simulink model "ADCS_orbiter_detumbling"  (R2022a)
settings: Solver=ode4  StartTime=0.0  StopTime=21085  FixedStep=0.1  MaxStep=1  RelTol=1e-8
values from neighbouring files (symbols this model uses):
  A_cube = 1    [Data_detumbling.m]    (also in main_orbiter_detumbling.m = 12.9)
  A_S2B = [1,0,0;0,-1,0;0,0,-1]    [Data_detumbling.m]
  alpha_x = deg2rad(6/3600)    [Data_detumbling.m]
  alpha_y = deg2rad(6/3600)    [Data_detumbling.m]
  alpha_z = deg2rad(40/3600)    [Data_detumbling.m]
  B_ast = pinv(B)    [Data_detumbling.m]
  ceps = cos(eps)    [Data_detumbling.m]    (also in main_orbiter_detumbling.m)
  F_max = 0.650    (= 0.65)    [Data_detumbling.m]    (also in main_orbiter_detumbling.m = 1.13)
  F_min = 0.160    (= 0.16)    [Data_detumbling.m]    (also in main_orbiter_detumbling.m = 0.19)
  J = [Jx,0,0 ... (first row only)    [Data_detumbling.m]    (also in DisturbanceEvaluation.m = {J_NSO; J_SO}; Thruster_sizing_2.m = diag([12043.36, 15990.19, 8547.84]); main_orbiter.m = J_SO; main_orbiter_detumbling.m = J_SO)
  k_dx = G*J(1,1)/max(diag(J))    [main_orbiter_detumbling.m]
  k_dy = G*J(2,2)/max(diag(J))    [main_orbiter_detumbling.m]
  k_dz = G*J(3,3)/max(diag(J))    [main_orbiter_detumbling.m]
  k_p = 0    [Data_detumbling.m]    (also in main_orbiter_detumbling.m)
  n1 = [1;0;0]    [Data_detumbling.m]    (also in main_orbiter_detumbling.m)
  n2 = [0;1;0]    [Data_detumbling.m]    (also in main_orbiter_detumbling.m)
  n3 = [0;0;1]    [Data_detumbling.m]    (also in main_orbiter_detumbling.m)
  n4 = -n1    [Data_detumbling.m]    (also in main_orbiter_detumbling.m)
  n5 = -n2    [Data_detumbling.m]    (also in main_orbiter_detumbling.m)
  n6 = -n3    [Data_detumbling.m]    (also in main_orbiter_detumbling.m)
  n_sun = 2*pi/(365.25*24*3600)    (= 1.99102127766e-07)    [Data_detumbling.m]    (also in main_orbiter_detumbling.m)
  P = F_e/c    [Data_detumbling.m]    (also in main_orbiter_detumbling.m)
  qbn0 = qrand./norm(qrand)    [main_orbiter.m]    (also in main_orbiter_detumbling.m)
  R = diag([lx_mb/2 ly_mb/2 lz_mb/2]) * [0  0  1  1  0  0 -1 -1 ... (first row only)    [Data_detumbling.m]    (also in main_orbiter_detumbling.m = 0.5*[-ly*cos(inc)              ly*cos(inc)            ly*cos)
  R_ast = pinv(R)    [Data_detumbling.m]    (also in main_orbiter_detumbling.m)
  r_i = r_cube * [n1,n2,n3,n4,n5,n6]    [Data_detumbling.m]    (also in main_orbiter_detumbling.m = [lx/2-cm_off_x  -cm_off_x       -cm_off_x        lx/2+cm_off)
  rho_d = 0.1    [Data_detumbling.m]    (also in main_orbiter_detumbling.m)
  rho_s = 0.5    [Data_detumbling.m]    (also in main_orbiter_detumbling.m)
  S_star1 = S_star1/norm(S_star1)    [Data_detumbling.m]
  S_star2 = S_star2/norm(S_star2)    [Data_detumbling.m]
  S_star3 = S_star3/norm(S_star3)    [Data_detumbling.m]
  S_star4 = S_star4/norm(S_star4)    [Data_detumbling.m]
  seps = sin(eps)    [Data_detumbling.m]    (also in main_orbiter_detumbling.m)
  sigma_ARW = deg2rad(0.001)    [main_orbiter_detumbling.m]
  state0 = [r_vec_new; v_vec_new]    [main_orbiter_detumbling.m]
  w = ones(length(R(1,:)),1)    [Data_detumbling.m]    (also in main_orbiter_detumbling.m)
  w_c = [0 0 0]'    [Data_detumbling.m]    (also in main_orbiter_detumbling.m)
  wb0 = 0.0001*rand(3, 1)    [main_orbiter.m]    (also in main_orbiter_detumbling.m = 0.1*rand(3, 1))
libraries: vrlib x8, matrix_library x1, simulink x1
(part 1 of 3)
settings Model: Creator=pietr  LastModifiedBy=26ele
settings DebuggingCC: UnconnectedInputMsg=warning  UnconnectedOutputMsg=warning  UnconnectedLineMsg=warning
settings RTWCC: DLArmComputeVersion=19.05

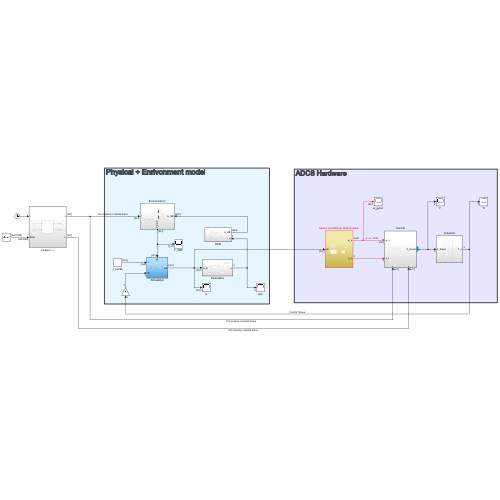
[thumbnail: Simulink's stored preview of the top-level diagram]
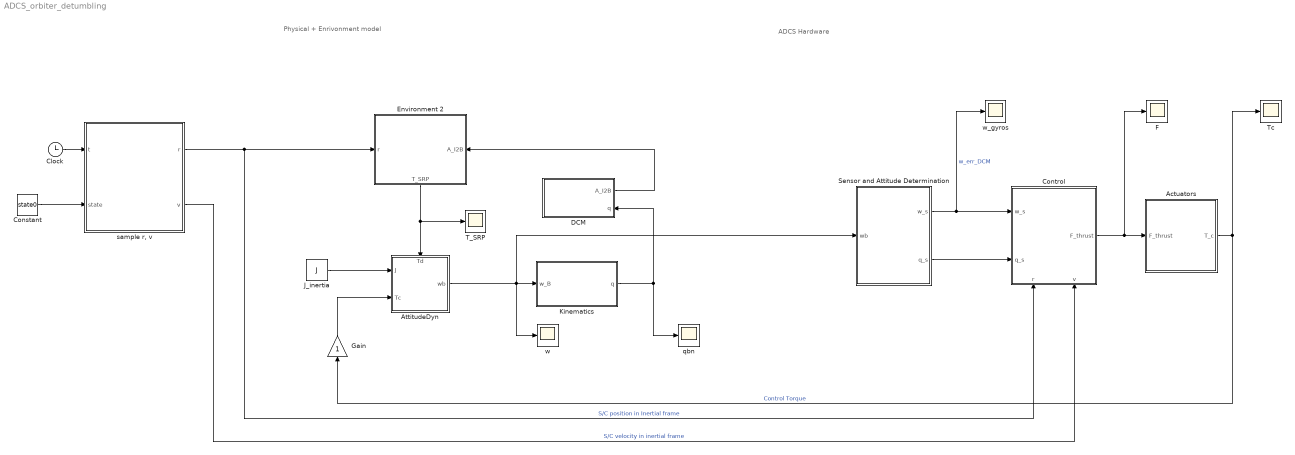
== system ADCS_orbiter_detumbling ==
  note: ADCS Hardware
  note: Physical + Enrivonment model
  Actuators : Subsystem
  AttitudeDyn : Subsystem
      settings: PortSchema="{\"entries\":[{\"content\":{\"sides\":[{\"content\":{\"connectorIds\":[\"In1\",\"In2\"]},\"type\":\"ConnectorPlacement.EquallySpacedRectSide\",\"uuid\":\"958d75f1-056c-4b4d-86fe-843bce156aeb\"},{\"content\":{\"connectorIds\":[\"Out1\"],\"side\":\"RIGHT\"},\"type\":\"ConnectorPlacement.EquallySpacedRectSide\",\"uuid\":\"65b3071b-d244-4f7f-a636-268af73b654f\"},{\"content\":{\"connectorIds\":[\"In3\"],\"side\":\"TOP\"},\"type\":\"ConnectorPlacement.EquallySpacedRectSide\",\"uuid\":\"8fd4fbc8-fd35-4e33-9d82-975bc389520f\"}]},\"type\":\"ConnectorPlacement.EquallySpacedConnector\",\"uuid\":\"8674dee0-aed3-475f-b5bf-17cea7319dbd\"}],\"packageUris\":[\"http://schema.mathworks.com/mf0/Connector/R2020b\"],\"version\":\"1.0\"}"
  Clock : Clock
  Constant : Constant  Value=state0
  Control : Subsystem
      settings: PortSchema="{\"entries\":[{\"content\":{\"sides\":[{\"content\":{\"connectorIds\":[\"In1\",\"In2\"]},\"type\":\"ConnectorPlacement.EquallySpacedRectSide\",\"uuid\":\"b61ecf6f-2766-421f-83dd-a531983edb9b\"},{\"content\":{\"connectorIds\":[\"Out1\"],\"side\":\"RIGHT\"},\"type\":\"ConnectorPlacement.EquallySpacedRectSide\",\"uuid\":\"105d38bf-fae8-4021-992b-3ab993bb750f\"},{\"content\":{\"connectorIds\":[\"In3\",\"In4\"],\"side\":\"TOP\"},\"type\":\"ConnectorPlacement.EquallySpacedRectSide\",\"uuid\":\"14e2d814-54f7-4199-8067-b878a77cfeec\"},{\"content\":{\"connectorIds\":[],\"side\":\"HIDDEN\"},\"type\":\"ConnectorPlacement.EquallySpacedRectSide\",\"uuid\":\"daf11c52-f465-40fd-b237-d971bdc47ecf\"}]},\"type\":\"ConnectorPlacement.EquallySpacedConnector\",\"uuid\":\"1c3e84f7-0d8e-475e-a711-13d0c4ce2024\"}],\"packageUris\":[\"http://schema.mathworks.com/mf0/Connector/R2020b\"],\"version\":\"1.0\"}"
  DCM : Subsystem
      settings: PortSchema="{\"entries\":[{\"content\":{\"sides\":[{\"content\":{\"connectorIds\":[]},\"type\":\"ConnectorPlacement.EquallySpacedRectSide\",\"uuid\":\"a2c03dcc-42ba-46b4-8766-9623140e285d\"},{\"content\":{\"connectorIds\":[\"Out1\",\"In1\"],\"side\":\"RIGHT\"},\"type\":\"ConnectorPlacement.EquallySpacedRectSide\",\"uuid\":\"181415b4-e06f-4a1b-bdae-77d0c2a7a22b\"},{\"content\":{\"connectorIds\":[],\"side\":\"TOP\"},\"type\":\"ConnectorPlacement.EquallySpacedRectSide\",\"uuid\":\"58a9c1ec-db17-43bd-920d-21c7ba7b5be3\"}]},\"type\":\"ConnectorPlacement.EquallySpacedConnector\",\"uuid\":\"76c9aeb0-6471-4cee-b641-2f0ff4597d57\"}],\"packageUris\":[\"http://schema.mathworks.com/mf0/Connector/R2020b\"],\"version\":\"1.0\"}"
  Environment 2 : Subsystem
      settings: PortSchema="{\"entries\":[{\"content\":{\"sides\":[{\"content\":{\"connectorIds\":[\"In1\"]},\"type\":\"ConnectorPlacement.EquallySpacedRectSide\",\"uuid\":\"bd1273ef-f007-48bf-a06f-e15d30a0e351\"},{\"content\":{\"connectorIds\":[\"In2\"],\"side\":\"RIGHT\"},\"type\":\"ConnectorPlacement.EquallySpacedRectSide\",\"uuid\":\"da98429c-d110-4330-bad5-271dcf5066c0\"},{\"content\":{\"connectorIds\":[],\"side\":\"TOP\"},\"type\":\"ConnectorPlacement.EquallySpacedRectSide\",\"uuid\":\"0aff5828-a0c0-41cd-a03e-5c9afd67cac4\"},{\"content\":{\"connectorIds\":[\"Out1\"],\"side\":\"BOTTOM\"},\"type\":\"ConnectorPlacement.EquallySpacedRectSide\",\"uuid\":\"8a284005-ec92-4f7e-b102-e371d7da8945\"}]},\"type\":\"ConnectorPlacement.EquallySpacedConnector\",\"uuid\":\"e9c1be51-430e-49aa-8c1f-f1d04716ab80\"}],\"packageUris\":[\"http://schema.mathworks.com/mf0/Connector/R2020b\"],\"version\":\"1.0\"}"
  F : Scope
  Gain : Gain
  J_inertia : Constant  Value=J  VectorParams1D=off
  Kinematics : Subsystem
  Sensor and Attitude Determination : Subsystem
  T_SRP : Scope
  Tc : Scope
  qbn : Scope
  "sample r, v" : Subsystem
  w : Scope
  w_gyros : Scope
  wires:
  Clock/1 -> "sample r, v"/1(t)
  Constant/1 -> "sample r, v"/2(state)
  "sample r, v"/1(r) -> Environment 2/1(r), Control/3(r)  "S/C position in Inertial frame"
  Kinematics/1(q) -> qbn/1, DCM/1(q)
  Sensor and Attitude Determination/1(w_s) -> w_gyros/1, Control/2(w_s)  "w_err_DCM"
  Sensor and Attitude Determination/2(q_s) -> Control/1(q_s)
  "sample r, v"/2(v) -> Control/4(v)  "S/C velocity in inertial frame"
  Control/1(F_thrust) -> F/1, Actuators/1(F_thrust)
  Actuators/1(T_c) -> Gain/1, Tc/1  "Control Torque"
  Gain/1 -> AttitudeDyn/2(Tc)
  AttitudeDyn/1(wb) -> w/1, Sensor and Attitude Determination/1(wb), Kinematics/1(w_B)
  J_inertia/1 -> AttitudeDyn/1(J)
  DCM/1(A_I2B) -> Environment 2/2(A_I2B)
  Environment 2/1(T_SRP) -> T_SRP/1, AttitudeDyn/3(Td)

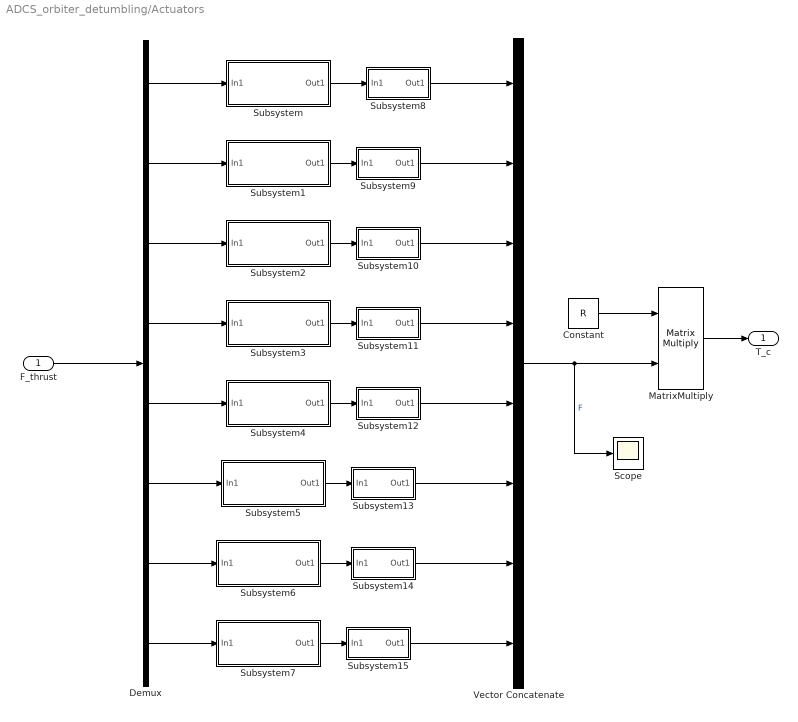
== system ADCS_orbiter_detumbling/Actuators ==
  F_thrust : Inport
  Constant : Constant  Value=R
  Demux : Demux  Outputs=8
  MatrixMultiply : Product  Multiplication=Matrix(*)
  Scope : Scope
  Subsystem : Subsystem
  Subsystem1 : Subsystem
  Subsystem10 : Subsystem
  Subsystem11 : Subsystem
  Subsystem12 : Subsystem
  Subsystem13 : Subsystem
  Subsystem14 : Subsystem
  Subsystem15 : Subsystem
  Subsystem2 : Subsystem
  Subsystem3 : Subsystem
  Subsystem4 : Subsystem
  Subsystem5 : Subsystem
  Subsystem6 : Subsystem
  Subsystem7 : Subsystem
  Subsystem8 : Subsystem
  Subsystem9 : Subsystem
  Vector Concatenate : Concatenate  NumInputs=8
  T_c : Outport
  wires:
  Constant/1 -> MatrixMultiply/1
  MatrixMultiply/1 -> T_c/1
  Vector Concatenate/1 -> Scope/1, MatrixMultiply/2  "F"
  Demux/8 -> Subsystem7/1(In1)
  Demux/7 -> Subsystem6/1(In1)
  F_thrust/1 -> Demux/1
  Demux/6 -> Subsystem5/1(In1)
  Demux/1 -> Subsystem/1(In1)
  Demux/2 -> Subsystem1/1(In1)
  Demux/3 -> Subsystem2/1(In1)
  Demux/4 -> Subsystem3/1(In1)
  Demux/5 -> Subsystem4/1(In1)
  Subsystem2/1(Out1) -> Subsystem10/1(In1)
  Subsystem3/1(Out1) -> Subsystem11/1(In1)
  Subsystem4/1(Out1) -> Subsystem12/1(In1)
  Subsystem5/1(Out1) -> Subsystem13/1(In1)
  Subsystem6/1(Out1) -> Subsystem14/1(In1)
  Subsystem7/1(Out1) -> Subsystem15/1(In1)
  Subsystem/1(Out1) -> Subsystem8/1(In1)
  Subsystem1/1(Out1) -> Subsystem9/1(In1)
  Subsystem15/1(Out1) -> Vector Concatenate/8
  Subsystem14/1(Out1) -> Vector Concatenate/7
  Subsystem13/1(Out1) -> Vector Concatenate/6
  Subsystem12/1(Out1) -> Vector Concatenate/5
  Subsystem11/1(Out1) -> Vector Concatenate/4
  Subsystem10/1(Out1) -> Vector Concatenate/3
  Subsystem9/1(Out1) -> Vector Concatenate/2
  Subsystem8/1(Out1) -> Vector Concatenate/1

== system ADCS_orbiter_detumbling/AttitudeDyn ==
  J : Inport
  Tc : Inport  Port=2
  Td : Inport  Port=3
  Cross Product1 : matrix_library/Cross Product
      settings: SourceProductBaseCode=SL
  Integrator : Integrator  InitialConditionSource=external
  Product : Product  Multiplication=Matrix(*)
  Product1 : Product  Inputs=/  Multiplication=Matrix(*)
  Sum : Sum  Inputs=-++
  To Workspace : ToWorkspace  VariableName=wb  SampleTime=-1
      settings: Save2DSignal=2-D array (concatenate along first dimension)
  wb0 : Constant  Value=wb0  VectorParams1D=off
  wbdot : Product  Multiplication=Matrix(*)
  wb : Outport
  wires:
  Integrator/1 -> wb/1, To Workspace/1, Product/2, Cross Product1/1
  Product/1 -> Cross Product1/2
  Cross Product1/1 -> Sum/1  "wcrossJw"
  J/1 -> Product1/1, Product/1
  wbdot/1 -> Integrator/1
  wb0/1 -> Integrator/2
  Tc/1 -> Sum/3
  Td/1 -> Sum/2
  Product1/1 -> wbdot/1
  Sum/1 -> wbdot/2

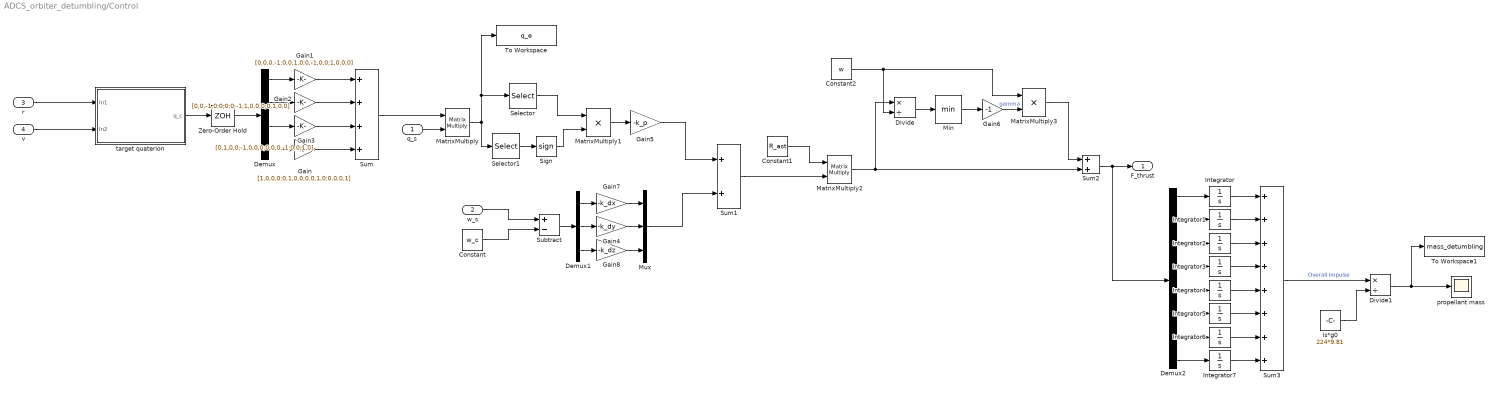
== system ADCS_orbiter_detumbling/Control ==
  q_s : Inport
  w_s : Inport  Port=2
  r : Inport  Port=3
  v : Inport  Port=4
  Constant : Constant  Value=w_c
  Constant1 : Constant  Value=R_ast
  Constant2 : Constant  Value=w
  Demux : Demux
  Demux1 : Demux  Outputs=3
  Demux2 : Demux  Outputs=8
  Divide : Product  Inputs=*/
  Divide1 : Product  Inputs=*/
  Gain : Gain  Gain=[1,0,0,0;0,1,0,0;0,0,1,0;0,0,0,1]
  Gain1 : Gain  Gain=[0,0,0,-1;0,0,1,0;0,-1,0,0;1,0,0,0]
  Gain2 : Gain  Gain=[0,0,-1,0;0,0,0,-1;1,0,0,0;0,1,0,0]
  Gain3 : Gain  Gain=[0,1,0,0;-1,0,0,0;0,0,0,-1;0,0,1,0]
  Gain4 : Gain  Gain=-k_dy
  Gain5 : Gain  Gain=-k_p
  Gain6 : Gain  Gain=-1
  Gain7 : Gain  Gain=-k_dx
  Gain8 : Gain  Gain=-k_dz
  Integrator{,1..7} (8 alike) : Integrator
  Is*g0 : Constant  Value=224*9.81
  MatrixMultiply : Product  Multiplication=Matrix(*)
  MatrixMultiply1 : Product
  MatrixMultiply2 : Product  Multiplication=Matrix(*)
  MatrixMultiply3 : Product
  Min : MinMax
  Mux : Mux  Inputs=3
  Selector : Selector  InputPortWidth=4  IndexOptions=Index vector (dialog)  Indices=[1 2 3]  OutputSizes=1
  Selector1 : Selector  InputPortWidth=4  IndexOptions=Index vector (dialog)  Indices=4  OutputSizes=1
  Sign : Signum
  Subtract : Sum  Inputs=+-
  Sum : Sum  Inputs=++++
  Sum1 : Sum
  Sum2 : Sum
  Sum3 : Sum  Inputs=++++++++
  To Workspace : ToWorkspace  VariableName=q_e  SaveFormat=Timeseries  SampleTime=-1
  To Workspace1 : ToWorkspace  VariableName=mass_detumbling  SampleTime=-1
  Zero-Order Hold : ZeroOrderHold  SampleTime=-1
  propellant mass : Scope
  target quaterion : Subsystem
  F_thrust : Outport
  wires:
  Selector1/1 -> Sign/1
  Constant/1 -> Subtract/2
  Subtract/1 -> Demux1/1
  w_s/1 -> Subtract/1
  MatrixMultiply/1 -> Selector1/1, Selector/1, To Workspace/1
  Zero-Order Hold/1 -> Demux/1
  target quaterion/1(q_c) -> Zero-Order Hold/1
  v/1 -> target quaterion/2(In2)
  r/1 -> target quaterion/1(In1)
  Gain5/1 -> Sum1/1
  Selector/1 -> MatrixMultiply1/1
  MatrixMultiply1/1 -> Gain5/1
  q_s/1 -> MatrixMultiply/2
  Sum/1 -> MatrixMultiply/1
  Gain/1 -> Sum/4
  Gain3/1 -> Sum/3
  Gain2/1 -> Sum/2
  Gain1/1 -> Sum/1
  Demux/2 -> Gain2/1
  Demux/3 -> Gain3/1
  Demux/1 -> Gain1/1
  Demux/4 -> Gain/1
  Sign/1 -> MatrixMultiply1/2
  Sum1/1 -> MatrixMultiply2/2
  Sum2/1 -> Demux2/1, F_thrust/1
  MatrixMultiply2/1 -> Divide/1, Sum2/2
  Divide/1 -> Min/1
  Constant1/1 -> MatrixMultiply2/1
  Gain6/1 -> MatrixMultiply3/2  "gamma"
  Min/1 -> Gain6/1
  Constant2/1 -> MatrixMultiply3/1, Divide/2
  MatrixMultiply3/1 -> Sum2/1
  Demux1/1 -> Gain7/1
  Gain7/1 -> Mux/1
  Demux1/2 -> Gain4/1
  Gain4/1 -> Mux/2
  Demux1/3 -> Gain8/1
  Gain8/1 -> Mux/3
  Mux/1 -> Sum1/2
  Integrator/1 -> Sum3/1
  Demux2/1 -> Integrator/1
  Demux2/2 -> Integrator1/1
  Demux2/8 -> Integrator7/1
  Demux2/7 -> Integrator6/1
  Demux2/6 -> Integrator5/1
  Demux2/5 -> Integrator4/1
  Demux2/4 -> Integrator3/1
  Demux2/3 -> Integrator2/1
  Integrator1/1 -> Sum3/2
  Integrator2/1 -> Sum3/3
  Integrator3/1 -> Sum3/4
  Integrator4/1 -> Sum3/5
  Integrator5/1 -> Sum3/6
  Integrator6/1 -> Sum3/7
  Integrator7/1 -> Sum3/8
  Sum3/1 -> Divide1/1  "Overall Impulse"
  Is*g0/1 -> Divide1/2
  Divide1/1 -> To Workspace1/1, propellant mass/1

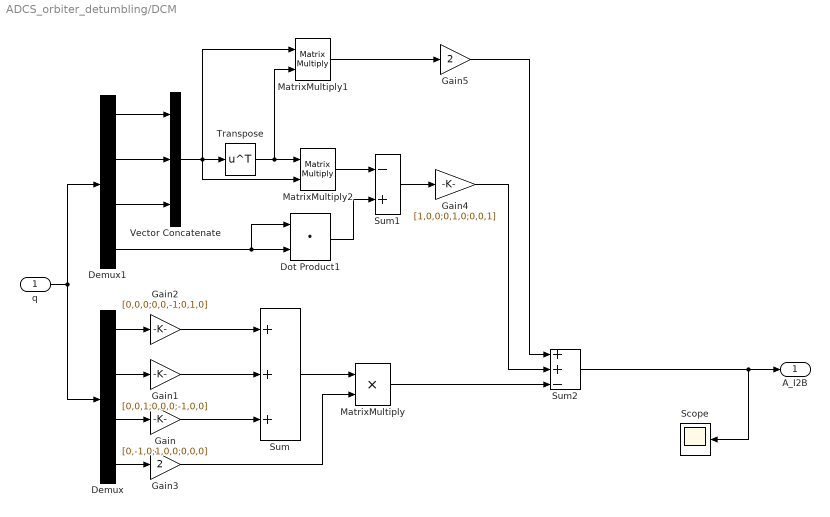
== system ADCS_orbiter_detumbling/DCM ==
  q : Inport
  Demux : Demux
  Demux1 : Demux
  Dot Product1 : DotProduct  OutDataTypeStr=Inherit: Inherit via internal rule
  Gain : Gain  Gain=[0,-1,0;1,0,0;0,0,0]
  Gain1 : Gain  Gain=[0,0,1;0,0,0;-1,0,0]
  Gain2 : Gain  Gain=[0,0,0;0,0,-1;0,1,0]
  Gain3 : Gain  Gain=2
  Gain4 : Gain  Gain=[1,0,0;0,1,0;0,0,1]
  Gain5 : Gain  Gain=2
  MatrixMultiply : Product
  MatrixMultiply1 : Product  Multiplication=Matrix(*)
  MatrixMultiply2 : Product  Multiplication=Matrix(*)
  Scope : Scope
  Sum : Sum  Inputs=+++
  Sum1 : Sum  Inputs=-+
  Sum2 : Sum  Inputs=++-
  Transpose : Math  Operator=transpose
  Vector Concatenate : Concatenate  NumInputs=3
  A_I2B : Outport
  wires:
  q/1 -> Demux/1, Demux1/1
  Demux/3 -> Gain/1
  Demux/2 -> Gain1/1
  Demux/1 -> Gain2/1
  Gain2/1 -> Sum/1
  Gain1/1 -> Sum/2
  Gain/1 -> Sum/3
  Demux/4 -> Gain3/1
  Gain3/1 -> MatrixMultiply/2
  Sum/1 -> MatrixMultiply/1
  Demux1/1 -> Vector Concatenate/1
  Demux1/2 -> Vector Concatenate/2
  Demux1/3 -> Vector Concatenate/3
  Vector Concatenate/1 -> MatrixMultiply1/1, MatrixMultiply2/2, Transpose/1
  Transpose/1 -> MatrixMultiply1/2, MatrixMultiply2/1
  Demux1/4 -> Dot Product1/1, Dot Product1/2
  MatrixMultiply2/1 -> Sum1/1
  Dot Product1/1 -> Sum1/2
  Sum1/1 -> Gain4/1
  MatrixMultiply/1 -> Sum2/3
  Gain4/1 -> Sum2/2
  MatrixMultiply1/1 -> Gain5/1
  Gain5/1 -> Sum2/1
  Sum2/1 -> Scope/1, A_I2B/1

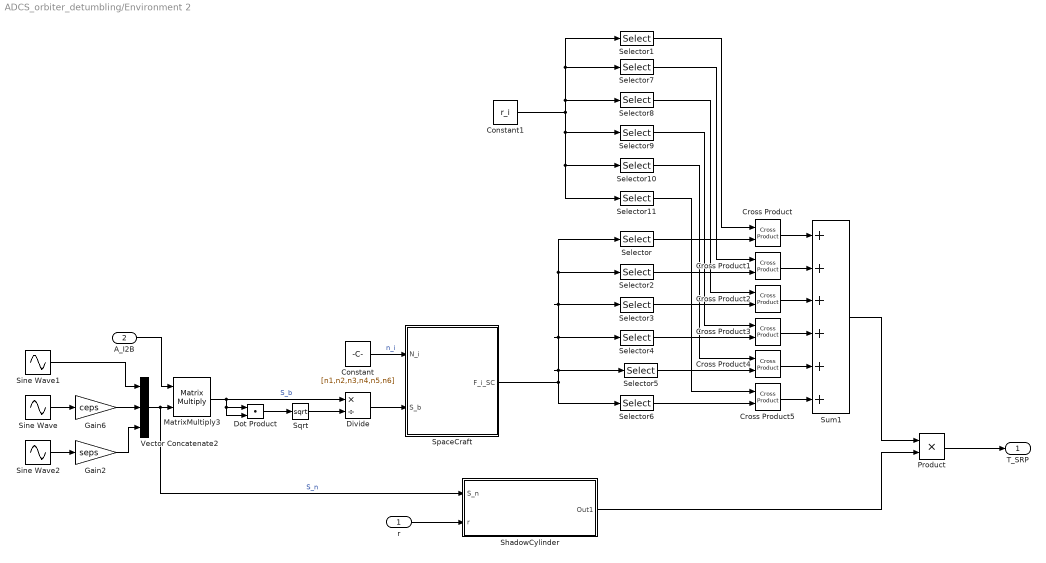
== system ADCS_orbiter_detumbling/Environment 2 ==
  r : Inport
  A_I2B : Inport  Port=2
  Constant : Constant  Value=[n1,n2,n3,n4,n5,n6]
  Constant1 : Constant  Value=r_i  VectorParams1D=off
  Cross Product{,1..5} (6 alike) : vrlib/Utilities/Cross Product
  Divide : Product  Inputs=*/
  Dot Product : DotProduct  OutDataTypeStr=Inherit: Inherit via internal rule
  Gain2 : Gain  Gain=seps
  Gain6 : Gain  Gain=ceps
  MatrixMultiply3 : Product  Multiplication=Matrix(*)
  Product : Product
  Selector : Selector  NumberOfDimensions=2  InputPortWidth=3  IndexOptions=Select all,Index vector (dialog)  Indices=1,1  OutputSizes=1,1
  Selector1 : Selector  NumberOfDimensions=2  InputPortWidth=3  IndexOptions=Select all,Index vector (dialog)  Indices=1,1  OutputSizes=1,1
  Selector10 : Selector  NumberOfDimensions=2  InputPortWidth=3  IndexOptions=Select all,Index vector (dialog)  Indices=5,5  OutputSizes=1,1
  Selector11 : Selector  NumberOfDimensions=2  InputPortWidth=3  IndexOptions=Select all,Index vector (dialog)  Indices=6,6  OutputSizes=1,1
  Selector2 : Selector  NumberOfDimensions=2  InputPortWidth=3  IndexOptions=Select all,Index vector (dialog)  Indices=2,2  OutputSizes=1,1
  Selector3 : Selector  NumberOfDimensions=2  InputPortWidth=3  IndexOptions=Select all,Index vector (dialog)  Indices=3,3  OutputSizes=1,1
  Selector4 : Selector  NumberOfDimensions=2  InputPortWidth=3  IndexOptions=Select all,Index vector (dialog)  Indices=4,4  OutputSizes=1,1
  Selector5 : Selector  NumberOfDimensions=2  InputPortWidth=3  IndexOptions=Select all,Index vector (dialog)  Indices=5,5  OutputSizes=1,1
  Selector6 : Selector  NumberOfDimensions=2  InputPortWidth=3  IndexOptions=Select all,Index vector (dialog)  Indices=6,6  OutputSizes=1,1
  Selector7 : Selector  NumberOfDimensions=2  InputPortWidth=3  IndexOptions=Select all,Index vector (dialog)  Indices=2,2  OutputSizes=1,1
  Selector8 : Selector  NumberOfDimensions=2  InputPortWidth=3  IndexOptions=Select all,Index vector (dialog)  Indices=3,3  OutputSizes=1,1
  Selector9 : Selector  NumberOfDimensions=2  InputPortWidth=3  IndexOptions=Select all,Index vector (dialog)  Indices=4,4  OutputSizes=1,1
  ShadowCylinder : Subsystem
  Sine Wave : Sin  Frequency=n_sun  SampleTime=0
  Sine Wave1 : Sin  Frequency=n_sun  Phase=pi/2  SampleTime=0
  Sine Wave2 : Sin  Frequency=n_sun  SampleTime=0
  SpaceCraft : Subsystem
  Sqrt : Sqrt
  Sum1 : Sum  Inputs=++++++
  Vector Concatenate2 : Concatenate  NumInputs=3
  T_SRP : Outport
  wires:
  SpaceCraft/1(F_i_SC) -> Selector5/1, Selector4/1, Selector3/1, Selector/1, Selector2/1, Selector6/1
  A_I2B/1 -> MatrixMultiply3/1
  Selector10/1 -> Cross Product4/1
  Gain2/1 -> Vector Concatenate2/3
  MatrixMultiply3/1 -> Divide/1, Dot Product/2, Dot Product/1  "S_b"
  Selector11/1 -> Cross Product5/1
  Cross Product2/1 -> Sum1/3
  Selector5/1 -> Cross Product4/2
  Selector9/1 -> Cross Product3/1
  Selector1/1 -> Cross Product/1
  Cross Product5/1 -> Sum1/6
  Sine Wave2/1 -> Gain2/1
  Dot Product/1 -> Sqrt/1
  Cross Product4/1 -> Sum1/5
  Selector6/1 -> Cross Product5/2
  Cross Product3/1 -> Sum1/4
  Selector4/1 -> Cross Product3/2
  Cross Product/1 -> Sum1/1
  Constant/1 -> SpaceCraft/1(N_i)  "n_i"
  Divide/1 -> SpaceCraft/2(S_b)
  Selector2/1 -> Cross Product1/2
  Selector8/1 -> Cross Product2/1
  Cross Product1/1 -> Sum1/2
  Selector3/1 -> Cross Product2/2
  Selector7/1 -> Cross Product1/1
  Selector/1 -> Cross Product/2
  Gain6/1 -> Vector Concatenate2/2
  Sine Wave/1 -> Gain6/1
  Sine Wave1/1 -> Vector Concatenate2/1
  Sum1/1 -> Product/1
  Sqrt/1 -> Divide/2
  Vector Concatenate2/1 -> ShadowCylinder/1(S_n), MatrixMultiply3/2  "S_n"
  r/1 -> ShadowCylinder/2(r)
  ShadowCylinder/1(Out1) -> Product/2
  Product/1 -> T_SRP/1
  Constant1/1 -> Selector1/1, Selector7/1, Selector8/1, Selector10/1, Selector11/1, Selector9/1

== system ADCS_orbiter_detumbling/Kinematics ==
  w_B : Inport
  Derivative : Derivative
  Quaternion : Subsystem
  To Workspace : ToWorkspace  VariableName=q  SampleTime=-1
  To Workspace1 : ToWorkspace  VariableName=w_B_dot  SaveFormat=Timeseries  SampleTime=-1
  q : Outport
  wires:
  Quaternion/1(q) -> To Workspace/1, q/1
  w_B/1 -> Derivative/1, Quaternion/1(w_B)
  Derivative/1 -> To Workspace1/1

== system ADCS_orbiter_detumbling/Sensor and Attitude Determination ==
  wb : Inport
  Gyroscope1 : Subsystem
  Star Trackers1 : Subsystem  Commented=on
  Subsystem2 : Subsystem
  Subsystem3 : Subsystem
  Subsystem4 : Subsystem
  Terminator : Terminator
  Terminator1 : Terminator
  w_s : Outport
  q_s : Outport  Port=2
  wires:
  Subsystem2/1(qerr) -> q_s/1
  Gyroscope1/1(w_GYR) -> w_s/1, Subsystem2/1(w_GYR)
  Star Trackers1/1(A_I2B_err) -> Subsystem4/1(A_I2B_err), Subsystem3/1(A_I2B_err)
  Subsystem3/1(qerr) -> Terminator1/1
  Subsystem4/1(w_err_DCM) -> Terminator/1
  wb/1 -> Gyroscope1/1(w)

== system ADCS_orbiter_detumbling/sample r, v ==
  t : Inport
  state : Inport  Port=2
  MATLAB Function : MATLAB Function  TreatAsAtomicUnit=on
  r : Outport
  v : Outport  Port=2
  wires:
  t/1 -> MATLAB Function/1(t)
  state/1 -> MATLAB Function/2(A)
  MATLAB Function/1(r) -> r/1
  MATLAB Function/2(v) -> v/1

== system ADCS_orbiter_detumbling/Actuators/Subsystem ==
  In1 : Inport
  Constant : Constant  Value=F_max
  Constant1 : Constant  Value=0
  If : If  IfExpression=u1 > F_max  ElseIfExpressions=u1<F_min
  If Action Subsystem : Subsystem  TreatAsAtomicUnit=on
  If Action Subsystem1 : Subsystem  TreatAsAtomicUnit=on
  If Action Subsystem2 : Subsystem  TreatAsAtomicUnit=on
  Merge : Merge  Inputs=3
  Out1 : Outport
  wires:
  In1/1 -> If/1, If Action Subsystem2/1(In1)
  If/1 -> If Action Subsystem/Action
  Constant/1 -> If Action Subsystem/1(In1)
  Constant1/1 -> If Action Subsystem1/1(In1)
  If/2 -> If Action Subsystem1/Action
  If/3 -> If Action Subsystem2/Action
  If Action Subsystem2/1(Out1) -> Merge/3
  If Action Subsystem/1(Out1) -> Merge/1
  If Action Subsystem1/1(Out1) -> Merge/2
  Merge/1 -> Out1/1

== system ADCS_orbiter_detumbling/Actuators/Subsystem1 ==
  In1 : Inport
  Constant : Constant  Value=F_max
  Constant1 : Constant  Value=0
  If : If  IfExpression=u1 > F_max  ElseIfExpressions=u1<F_min
  If Action Subsystem : Subsystem  TreatAsAtomicUnit=on
  If Action Subsystem1 : Subsystem  TreatAsAtomicUnit=on
  If Action Subsystem2 : Subsystem  TreatAsAtomicUnit=on
  Merge : Merge  Inputs=3
  Out1 : Outport
  wires:
  In1/1 -> If Action Subsystem2/1(In1), If/1
  If/1 -> If Action Subsystem/Action
  Constant/1 -> If Action Subsystem/1(In1)
  Constant1/1 -> If Action Subsystem1/1(In1)
  If/2 -> If Action Subsystem1/Action
  If/3 -> If Action Subsystem2/Action
  If Action Subsystem2/1(Out1) -> Merge/3
  If Action Subsystem/1(Out1) -> Merge/1
  If Action Subsystem1/1(Out1) -> Merge/2
  Merge/1 -> Out1/1

== system ADCS_orbiter_detumbling/Actuators/Subsystem10 ==
  In1 : Inport
  Delay : Delay  DelayLength=1
  Delay1 : Delay
  If : If
  If Action Subsystem : Subsystem  TreatAsAtomicUnit=on
  If Action Subsystem1 : Subsystem  TreatAsAtomicUnit=on
  Merge : Merge
  Out1 : Outport
  wires:
  In1/1 -> Delay/1, Delay1/1, If Action Subsystem1/1(In1), If Action Subsystem/1(In1), If/1
  If/1 -> If Action Subsystem/Action
  If/2 -> If Action Subsystem1/Action
  If Action Subsystem/1(Out2) -> Merge/1  "u"
  If Action Subsystem1/1(Out1) -> Merge/2  "u"
  Merge/1 -> Out1/1
  Delay/1 -> If Action Subsystem1/2(Input)
  Delay1/1 -> If Action Subsystem1/3(Input1)

== system ADCS_orbiter_detumbling/Actuators/Subsystem11 ==
  In1 : Inport
  Delay : Delay  DelayLength=1
  Delay1 : Delay
  If : If
  If Action Subsystem : Subsystem  TreatAsAtomicUnit=on
  If Action Subsystem1 : Subsystem  TreatAsAtomicUnit=on
  Merge : Merge
  Out1 : Outport
  wires:
  Delay1/1 -> If Action Subsystem1/3(Input1)
  Delay/1 -> If Action Subsystem1/2(Input)
  Merge/1 -> Out1/1
  If Action Subsystem1/1(Out1) -> Merge/2  "u"
  If Action Subsystem/1(Out2) -> Merge/1  "u"
  If/2 -> If Action Subsystem1/Action
  If/1 -> If Action Subsystem/Action
  In1/1 -> If/1, If Action Subsystem/1(In1), If Action Subsystem1/1(In1), Delay1/1, Delay/1

== system ADCS_orbiter_detumbling/Actuators/Subsystem12 ==
  In1 : Inport
  Delay : Delay  DelayLength=1
  Delay1 : Delay
  If : If
  If Action Subsystem : Subsystem  TreatAsAtomicUnit=on
  If Action Subsystem1 : Subsystem  TreatAsAtomicUnit=on
  Merge : Merge
  Out1 : Outport
  wires:
  In1/1 -> Delay/1, Delay1/1, If Action Subsystem1/1(In1), If Action Subsystem/1(In1), If/1
  If/1 -> If Action Subsystem/Action
  If/2 -> If Action Subsystem1/Action
  If Action Subsystem/1(Out2) -> Merge/1  "u"
  If Action Subsystem1/1(Out1) -> Merge/2  "u"
  Merge/1 -> Out1/1
  Delay/1 -> If Action Subsystem1/2(Input)
  Delay1/1 -> If Action Subsystem1/3(Input1)

== system ADCS_orbiter_detumbling/Actuators/Subsystem13 ==
  In1 : Inport
  Delay : Delay  DelayLength=1
  Delay1 : Delay
  If : If
  If Action Subsystem : Subsystem  TreatAsAtomicUnit=on
  If Action Subsystem1 : Subsystem  TreatAsAtomicUnit=on
  Merge : Merge
  Scope : Scope  NumInputPorts=2
  Out1 : Outport
  wires:
  Delay1/1 -> If Action Subsystem1/3(Input1)
  Delay/1 -> If Action Subsystem1/2(Input)
  Merge/1 -> Scope/2, Out1/1
  If Action Subsystem1/1(Out1) -> Merge/2  "u"
  If Action Subsystem/1(Out2) -> Merge/1  "u"
  If/2 -> If Action Subsystem1/Action
  If/1 -> If Action Subsystem/Action
  In1/1 -> If/1, Scope/1, If Action Subsystem/1(In1), If Action Subsystem1/1(In1), Delay1/1, Delay/1

== system ADCS_orbiter_detumbling/Actuators/Subsystem14 ==
  In1 : Inport
  Delay : Delay  DelayLength=1
  Delay1 : Delay
  If : If
  If Action Subsystem : Subsystem  TreatAsAtomicUnit=on
  If Action Subsystem1 : Subsystem  TreatAsAtomicUnit=on
  Merge : Merge
  Scope : Scope  NumInputPorts=2
  Out1 : Outport
  wires:
  In1/1 -> Delay/1, Delay1/1, If Action Subsystem1/1(In1), Scope/1, If Action Subsystem/1(In1), If/1
  If/1 -> If Action Subsystem/Action
  If/2 -> If Action Subsystem1/Action
  If Action Subsystem/1(Out2) -> Merge/1  "u"
  If Action Subsystem1/1(Out1) -> Merge/2  "u"
  Merge/1 -> Scope/2, Out1/1
  Delay/1 -> If Action Subsystem1/2(Input)
  Delay1/1 -> If Action Subsystem1/3(Input1)

== system ADCS_orbiter_detumbling/Actuators/Subsystem15 ==
  In1 : Inport
  Delay : Delay  DelayLength=1
  Delay1 : Delay
  If : If
  If Action Subsystem : Subsystem  TreatAsAtomicUnit=on
  If Action Subsystem1 : Subsystem  TreatAsAtomicUnit=on
  Merge : Merge
  Out1 : Outport
  wires:
  Delay1/1 -> If Action Subsystem1/3(Input1)
  Delay/1 -> If Action Subsystem1/2(Input)
  Merge/1 -> Out1/1
  If Action Subsystem1/1(Out1) -> Merge/2  "u"
  If Action Subsystem/1(Out2) -> Merge/1  "u"
  If/2 -> If Action Subsystem1/Action
  If/1 -> If Action Subsystem/Action
  In1/1 -> If/1, If Action Subsystem/1(In1), If Action Subsystem1/1(In1), Delay1/1, Delay/1

== system ADCS_orbiter_detumbling/Actuators/Subsystem2 ==
  In1 : Inport
  Constant : Constant  Value=F_max
  Constant1 : Constant  Value=0
  If : If  IfExpression=u1 > F_max  ElseIfExpressions=u1<F_min
  If Action Subsystem : Subsystem  TreatAsAtomicUnit=on
  If Action Subsystem1 : Subsystem  TreatAsAtomicUnit=on
  If Action Subsystem2 : Subsystem  TreatAsAtomicUnit=on
  Merge : Merge  Inputs=3
  Out1 : Outport
  wires:
  Merge/1 -> Out1/1
  If Action Subsystem1/1(Out1) -> Merge/2
  If Action Subsystem/1(Out1) -> Merge/1
  If Action Subsystem2/1(Out1) -> Merge/3
  If/3 -> If Action Subsystem2/Action
  If/2 -> If Action Subsystem1/Action
  Constant1/1 -> If Action Subsystem1/1(In1)
  Constant/1 -> If Action Subsystem/1(In1)
  If/1 -> If Action Subsystem/Action
  In1/1 -> If/1, If Action Subsystem2/1(In1)

== system ADCS_orbiter_detumbling/Actuators/Subsystem3 ==
  In1 : Inport
  Constant : Constant  Value=F_max
  Constant1 : Constant  Value=0
  If : If  IfExpression=u1 > F_max  ElseIfExpressions=u1<F_min
  If Action Subsystem : Subsystem  TreatAsAtomicUnit=on
  If Action Subsystem1 : Subsystem  TreatAsAtomicUnit=on
  If Action Subsystem2 : Subsystem  TreatAsAtomicUnit=on
  Merge : Merge  Inputs=3
  Out1 : Outport
  wires:
  In1/1 -> If Action Subsystem2/1(In1), If/1
  If/1 -> If Action Subsystem/Action
  Constant/1 -> If Action Subsystem/1(In1)
  Constant1/1 -> If Action Subsystem1/1(In1)
  If/2 -> If Action Subsystem1/Action
  If/3 -> If Action Subsystem2/Action
  If Action Subsystem2/1(Out1) -> Merge/3
  If Action Subsystem/1(Out1) -> Merge/1
  If Action Subsystem1/1(Out1) -> Merge/2
  Merge/1 -> Out1/1

== system ADCS_orbiter_detumbling/Actuators/Subsystem4 ==
  In1 : Inport
  Constant : Constant  Value=F_max
  Constant1 : Constant  Value=0
  If : If  IfExpression=u1 > F_max  ElseIfExpressions=u1<F_min
  If Action Subsystem : Subsystem  TreatAsAtomicUnit=on
  If Action Subsystem1 : Subsystem  TreatAsAtomicUnit=on
  If Action Subsystem2 : Subsystem  TreatAsAtomicUnit=on
  Merge : Merge  Inputs=3
  Out1 : Outport
  wires:
  Merge/1 -> Out1/1
  If Action Subsystem1/1(Out1) -> Merge/2
  If Action Subsystem/1(Out1) -> Merge/1
  If Action Subsystem2/1(Out1) -> Merge/3
  If/3 -> If Action Subsystem2/Action
  If/2 -> If Action Subsystem1/Action
  Constant1/1 -> If Action Subsystem1/1(In1)
  Constant/1 -> If Action Subsystem/1(In1)
  If/1 -> If Action Subsystem/Action
  In1/1 -> If/1, If Action Subsystem2/1(In1)

== system ADCS_orbiter_detumbling/Actuators/Subsystem5 ==
  In1 : Inport
  Constant : Constant  Value=F_max
  Constant1 : Constant  Value=0
  If : If  IfExpression=u1 > F_max  ElseIfExpressions=u1<F_min
  If Action Subsystem : Subsystem  TreatAsAtomicUnit=on
  If Action Subsystem1 : Subsystem  TreatAsAtomicUnit=on
  If Action Subsystem2 : Subsystem  TreatAsAtomicUnit=on
  Merge : Merge  Inputs=3
  Out1 : Outport
  wires:
  In1/1 -> If Action Subsystem2/1(In1), If/1
  If/1 -> If Action Subsystem/Action
  Constant/1 -> If Action Subsystem/1(In1)
  Constant1/1 -> If Action Subsystem1/1(In1)
  If/2 -> If Action Subsystem1/Action
  If/3 -> If Action Subsystem2/Action
  If Action Subsystem2/1(Out1) -> Merge/3
  If Action Subsystem/1(Out1) -> Merge/1
  If Action Subsystem1/1(Out1) -> Merge/2
  Merge/1 -> Out1/1

== system ADCS_orbiter_detumbling/Actuators/Subsystem6 ==
  In1 : Inport
  Constant : Constant  Value=F_max
  Constant1 : Constant  Value=0
  If : If  IfExpression=u1 > F_max  ElseIfExpressions=u1<F_min
  If Action Subsystem : Subsystem  TreatAsAtomicUnit=on
  If Action Subsystem1 : Subsystem  TreatAsAtomicUnit=on
  If Action Subsystem2 : Subsystem  TreatAsAtomicUnit=on
  Merge : Merge  Inputs=3
  Out1 : Outport
  wires:
  Merge/1 -> Out1/1
  If Action Subsystem1/1(Out1) -> Merge/2
  If Action Subsystem/1(Out1) -> Merge/1
  If Action Subsystem2/1(Out1) -> Merge/3
  If/3 -> If Action Subsystem2/Action
  If/2 -> If Action Subsystem1/Action
  Constant1/1 -> If Action Subsystem1/1(In1)
  Constant/1 -> If Action Subsystem/1(In1)
  If/1 -> If Action Subsystem/Action
  In1/1 -> If/1, If Action Subsystem2/1(In1)

== system ADCS_orbiter_detumbling/Actuators/Subsystem7 ==
  In1 : Inport
  Constant : Constant  Value=F_max
  Constant1 : Constant  Value=0
  If : If  IfExpression=u1 > F_max  ElseIfExpressions=u1<F_min
  If Action Subsystem : Subsystem  TreatAsAtomicUnit=on
  If Action Subsystem1 : Subsystem  TreatAsAtomicUnit=on
  If Action Subsystem2 : Subsystem  TreatAsAtomicUnit=on
  Merge : Merge  Inputs=3
  Out1 : Outport
  wires:
  In1/1 -> If Action Subsystem2/1(In1), If/1
  If/1 -> If Action Subsystem/Action
  Constant/1 -> If Action Subsystem/1(In1)
  Constant1/1 -> If Action Subsystem1/1(In1)
  If/2 -> If Action Subsystem1/Action
  If/3 -> If Action Subsystem2/Action
  If Action Subsystem2/1(Out1) -> Merge/3
  If Action Subsystem/1(Out1) -> Merge/1
  If Action Subsystem1/1(Out1) -> Merge/2
  Merge/1 -> Out1/1

== system ADCS_orbiter_detumbling/Actuators/Subsystem8 ==
  In1 : Inport
  Delay : Delay  DelayLength=1
  Delay1 : Delay
  If : If
  If Action Subsystem : Subsystem  TreatAsAtomicUnit=on
  If Action Subsystem1 : Subsystem  TreatAsAtomicUnit=on
  Merge : Merge
  Out1 : Outport
  wires:
  In1/1 -> Delay/1, Delay1/1, If Action Subsystem1/1(In1), If Action Subsystem/1(In1), If/1
  If/1 -> If Action Subsystem/Action
  If/2 -> If Action Subsystem1/Action
  If Action Subsystem/1(Out2) -> Merge/1  "u"
  If Action Subsystem1/1(Out1) -> Merge/2  "u"
  Merge/1 -> Out1/1
  Delay/1 -> If Action Subsystem1/2(Input)
  Delay1/1 -> If Action Subsystem1/3(Input1)

== system ADCS_orbiter_detumbling/Actuators/Subsystem9 ==
  In1 : Inport
  Delay : Delay  DelayLength=1
  Delay1 : Delay
  If : If
  If Action Subsystem : Subsystem  TreatAsAtomicUnit=on
  If Action Subsystem1 : Subsystem  TreatAsAtomicUnit=on
  Merge : Merge
  Out1 : Outport
  wires:
  Delay1/1 -> If Action Subsystem1/3(Input1)
  Delay/1 -> If Action Subsystem1/2(Input)
  Merge/1 -> Out1/1
  If Action Subsystem1/1(Out1) -> Merge/2  "u"
  If Action Subsystem/1(Out2) -> Merge/1  "u"
  If/2 -> If Action Subsystem1/Action
  If/1 -> If Action Subsystem/Action
  In1/1 -> If/1, If Action Subsystem/1(In1), If Action Subsystem1/1(In1), Delay1/1, Delay/1

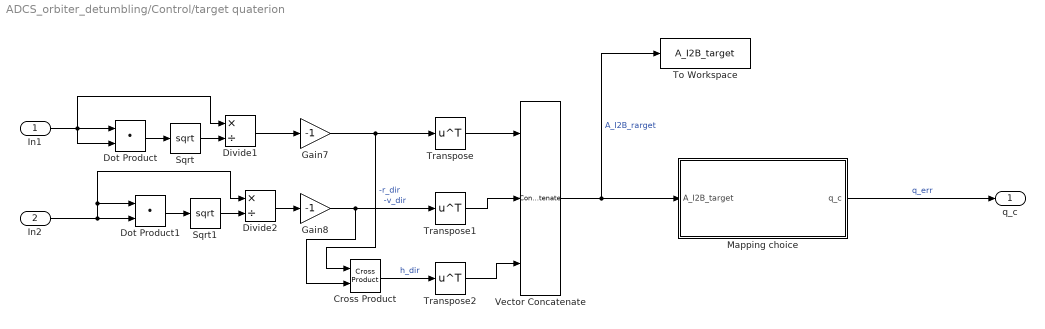
== system ADCS_orbiter_detumbling/Control/target quaterion ==
  In1 : Inport
  In2 : Inport  Port=2
  Cross Product : vrlib/Utilities/Cross Product
  Divide1 : Product  Inputs=*/
  Divide2 : Product  Inputs=*/
  Dot Product : DotProduct  OutDataTypeStr=Inherit: Inherit via internal rule
  Dot Product1 : DotProduct  OutDataTypeStr=Inherit: Inherit via internal rule
  Gain7 : Gain  Gain=-1
  Gain8 : Gain  Gain=-1
  Mapping choice : Subsystem
  Sqrt : Sqrt
  Sqrt1 : Sqrt
  To Workspace : ToWorkspace  VariableName=A_I2B_target  SampleTime=-1
  Transpose : Math  Operator=transpose
  Transpose1 : Math  Operator=transpose
  Transpose2 : Math  Operator=transpose
  Vector Concatenate : Concatenate  NumInputs=3  Mode=Multidimensional array
  q_c : Outport
  wires:
  Mapping choice/1(q_c) -> q_c/1  "q_err"
  Sqrt/1 -> Divide1/2
  Transpose2/1 -> Vector Concatenate/3
  Cross Product/1 -> Transpose2/1  "h_dir"
  Dot Product1/1 -> Sqrt1/1
  Divide2/1 -> Gain8/1
  Sqrt1/1 -> Divide2/2
  Divide1/1 -> Gain7/1
  Vector Concatenate/1 -> To Workspace/1, Mapping choice/1(A_I2B_target)  "A_I2B_rarget"
  Transpose1/1 -> Vector Concatenate/2
  In1/1 -> Dot Product/2, Divide1/1, Dot Product/1
  Gain7/1 -> Transpose/1, Cross Product/1  "-r_dir"
  Dot Product/1 -> Sqrt/1
  Transpose/1 -> Vector Concatenate/1
  In2/1 -> Dot Product1/2, Divide2/1, Dot Product1/1
  Gain8/1 -> Transpose1/1, Cross Product/2  "-v_dir"

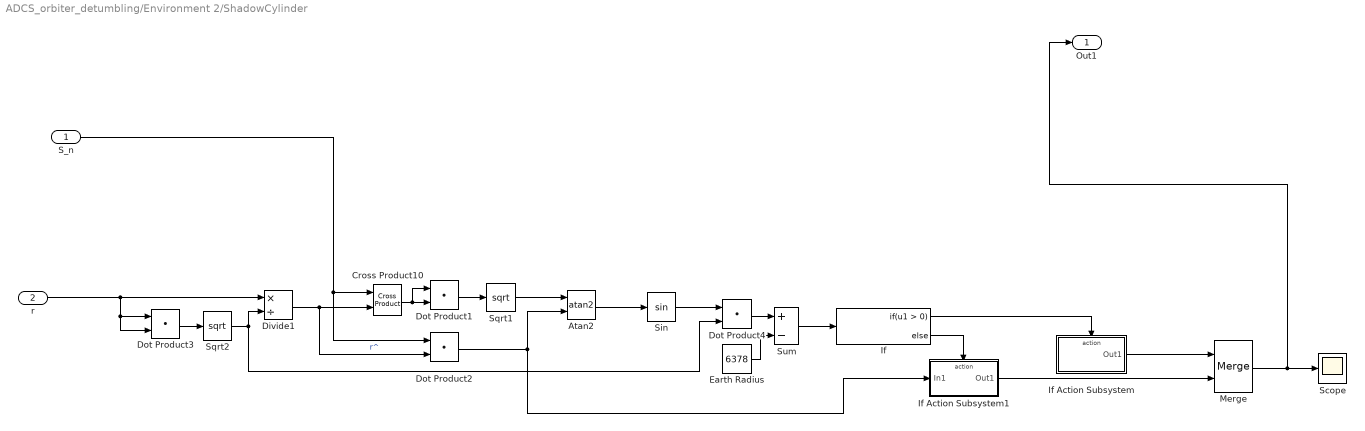
== system ADCS_orbiter_detumbling/Environment 2/ShadowCylinder ==
  S_n : Inport
  r : Inport  Port=2
  Atan2 : Trigonometry  Operator=atan2  OutputSignalType=real
  Cross Product10 : vrlib/Utilities/Cross Product
  Divide1 : Product  Inputs=*/
  Dot Product{1..4} (4 alike) : DotProduct  OutDataTypeStr=Inherit: Inherit via internal rule
  Earth Radius : Constant  Value=6378
  If : If
  If Action Subsystem : Subsystem  TreatAsAtomicUnit=on
  If Action Subsystem1 : Subsystem  TreatAsAtomicUnit=on
  Merge : Merge
  Scope : Scope
  Sin : Trigonometry
  Sqrt1 : Sqrt
  Sqrt2 : Sqrt
  Sum : Sum  Inputs=+-
  Out1 : Outport
  wires:
  Sqrt1/1 -> Atan2/1
  Cross Product10/1 -> Dot Product1/1, Dot Product1/2
  Dot Product1/1 -> Sqrt1/1
  Sqrt2/1 -> Dot Product4/2, Divide1/2
  If/2 -> If Action Subsystem1/Action
  Divide1/1 -> Dot Product2/2, Cross Product10/2  "r^"
  Atan2/1 -> Sin/1
  r/1 -> Divide1/1, Dot Product3/1, Dot Product3/2
  Dot Product2/1 -> If Action Subsystem1/1(In1), Atan2/2
  S_n/1 -> Dot Product2/1, Cross Product10/1
  Sum/1 -> If/1
  Dot Product4/1 -> Sum/1
  If/1 -> If Action Subsystem/Action
  If Action Subsystem/1(Out1) -> Merge/1
  Earth Radius/1 -> Sum/2
  Sin/1 -> Dot Product4/1
  Dot Product3/1 -> Sqrt2/1
  If Action Subsystem1/1(Out1) -> Merge/2
  Merge/1 -> Out1/1, Scope/1

== system ADCS_orbiter_detumbling/Environment 2/SpaceCraft ==
  N_i : Inport
  S_b : Inport  Port=2
  Constant : Constant  Value=2/3*rho_d
  Gain : Gain  Gain=1-rho_s
  Gain1 : Gain  Gain=2*rho_s
  Gain2 : Gain  Gain=-P*A_cube
  Gain3 : Gain  Gain=[1,1,1,1,1,1]
  MatrixMultiply : Product  Multiplication=Matrix(*)
  MatrixMultiply1 : Product  Multiplication=Matrix(*)
  MatrixMultiply2 : Product  Multiplication=Matrix(*)
  Sum : Sum
  Sum1 : Sum
  Transpose : Math  Operator=transpose
  Transpose2 : Math  Operator=transpose
  Zero_If_Negative : Subsystem
  F_i_SC : Outport
  wires:
  N_i/1 -> MatrixMultiply1/1, MatrixMultiply/2  "N_i"
  S_b/1 -> Gain/1, Transpose2/1
  MatrixMultiply/1 -> Gain1/1, Zero_If_Negative/1(In1)  "S_bN_i"
  Gain2/1 -> F_i_SC/1  "F_i_SC"
  Sum/1 -> MatrixMultiply1/2
  MatrixMultiply1/1 -> Sum1/2
  Gain/1 -> Sum1/1
  Sum1/1 -> MatrixMultiply2/1
  MatrixMultiply2/1 -> Gain2/1
  Transpose2/1 -> MatrixMultiply/1
  Gain1/1 -> Transpose/1
  Constant/1 -> Gain3/1
  Gain3/1 -> Sum/2
  Transpose/1 -> Sum/1
  Zero_If_Negative/1(Out1) -> MatrixMultiply2/2

== system ADCS_orbiter_detumbling/Kinematics/Quaternion ==
  w_B : Inport
  Demux : Demux  Outputs=3
  Divide : Product  Inputs=*/
  Dot Product : DotProduct  OutDataTypeStr=Inherit: Inherit via internal rule
  Gain2 : Gain  Gain=1/2
  Gain3 : Gain  Gain=[0,0,0,1;0,0,1,0;0,-1,0,0;-1,0,0,0]
  Gain4 : Gain  Gain=[0,0,-1,0;0,0,0,1;1,0,0,0;0,-1,0,0]
  Gain5 : Gain  Gain=[0,1,0,0;-1,0,0,0;0,0,0,1;0,0,-1,0]
  Integrator1 : Integrator  InitialCondition=qbn0
  MatrixMultiply : Product  Multiplication=Matrix(*)
  Sqrt : Sqrt
  Sum : Sum  Inputs=+++
  q : Outport
  wires:
  Gain4/1 -> Sum/2
  w_B/1 -> Demux/1
  Gain5/1 -> Sum/3
  Demux/2 -> Gain4/1
  Demux/1 -> Gain3/1
  Integrator1/1 -> Dot Product/2, Dot Product/1, Divide/1, q/1  "q"
  Gain3/1 -> Sum/1
  Demux/3 -> Gain5/1
  Gain2/1 -> Integrator1/1
  Sum/1 -> MatrixMultiply/1  "OMEGA"
  Divide/1 -> MatrixMultiply/2  "q"
  MatrixMultiply/1 -> Gain2/1
  Dot Product/1 -> Sqrt/1
  Sqrt/1 -> Divide/2

== system ADCS_orbiter_detumbling/Sensor and Attitude Determination/Gyroscope1 ==
  w : Inport
  Add : Sum  Inputs=+++
  Integrator2 : Integrator
  Mux : Mux  Inputs=3
  Mux1 : Mux  Inputs=3
  Random Number{,1..5} (6 alike) : RandomNumber  Variance=sigma_ARW^2  Seed=20  SampleTime=0.1
  Zero-Order Hold : ZeroOrderHold  SampleTime=-1
  w_GYR : Outport
  wires:
  Random Number5/1 -> Mux/3
  Zero-Order Hold/1 -> w_GYR/1
  Add/1 -> Zero-Order Hold/1
  w/1 -> Add/1
  Integrator2/1 -> Add/3
  Mux1/1 -> Add/2  "w_ARW"
  Random Number/1 -> Mux1/1
  Random Number3/1 -> Mux1/3
  Random Number2/1 -> Mux1/2
  Random Number1/1 -> Mux/1
  Mux/1 -> Integrator2/1  "w_RRW"
  Random Number4/1 -> Mux/2

== system ADCS_orbiter_detumbling/Sensor and Attitude Determination/Star Trackers1 ==
  A_I2B : Inport
  Constant4 : Constant  Value=B_ast
  Gain{1..3,14} (4 alike) : Gain  Gain=A_S2B  Multiplication=Matrix(K*u)
  MatrixMultiply : Product  Multiplication=Matrix(*)
  Sensor : Subsystem
  Vector Concatenate1 : Concatenate  NumInputs=4  Mode=Multidimensional array  ConcatenateDimension=2
  A_I2B_err : Outport
  wires:
  Sensor/4(Out4) -> Gain3/1
  Sensor/2(Out2) -> Gain1/1
  Gain3/1 -> Vector Concatenate1/4  "S4_B_err"
  Constant4/1 -> MatrixMultiply/2
  Sensor/3(Out3) -> Gain2/1
  Gain14/1 -> Vector Concatenate1/1  "S1_B_err"
  Gain1/1 -> Vector Concatenate1/2  "S2_B_err"
  Gain2/1 -> Vector Concatenate1/3  "S3_B_err"
  Sensor/1(Out1) -> Gain14/1
  Vector Concatenate1/1 -> MatrixMultiply/1
  A_I2B/1 -> Sensor/1(A_I2B)
  MatrixMultiply/1 -> A_I2B_err/1  "A_I2B_err"

== system ADCS_orbiter_detumbling/Sensor and Attitude Determination/Subsystem2 ==
  w_GYR : Inport
  Demux : Demux  Outputs=3
  Divide : Product  Inputs=*/
  Dot Product : DotProduct  OutDataTypeStr=Inherit: Inherit via internal rule
  Gain2 : Gain  Gain=1/2
  Gain3 : Gain  Gain=[0,0,0,1;0,0,1,0;0,-1,0,0;-1,0,0,0]
  Gain4 : Gain  Gain=[0,0,-1,0;0,0,0,1;1,0,0,0;0,-1,0,0]
  Gain5 : Gain  Gain=[0,1,0,0;-1,0,0,0;0,0,0,1;0,0,-1,0]
  Integrator1 : Integrator  InitialCondition=qbn0
  MatrixMultiply : Product  Multiplication=Matrix(*)
  Sqrt : Sqrt
  Sum : Sum  Inputs=+++
  qerr : Outport
  wires:
  Sqrt/1 -> Divide/2
  Gain2/1 -> Integrator1/1
  Dot Product/1 -> Sqrt/1
  Gain3/1 -> Sum/1
  MatrixMultiply/1 -> Gain2/1
  Sum/1 -> MatrixMultiply/1  "OMEGA"
  Divide/1 -> MatrixMultiply/2  "q"
  Demux/3 -> Gain5/1
  Demux/2 -> Gain4/1
  w_GYR/1 -> Demux/1
  Integrator1/1 -> qerr/1, Dot Product/2, Dot Product/1, Divide/1  "q"
  Demux/1 -> Gain3/1
  Gain5/1 -> Sum/3
  Gain4/1 -> Sum/2

== system ADCS_orbiter_detumbling/Sensor and Attitude Determination/Subsystem3 ==
  A_I2B_err : Inport
  Constant1 : Constant  Commented=on
  From q4 : Subsystem  Commented=on
  Gain2 : Gain  Commented=on  Gain=1/2
  Mapping choice : Subsystem
  Selector : Selector  Commented=on  NumberOfDimensions=2  InputPortWidth=3  IndexOptions=Index vector (dialog),Index vector (dialog)  Indices=1,1  OutputSizes=1,1
  Selector10 : Selector  Commented=on  NumberOfDimensions=2  InputPortWidth=3  IndexOptions=Index vector (dialog),Index vector (dialog)  Indices=2,2  OutputSizes=1,1
  Selector11 : Selector  Commented=on  NumberOfDimensions=2  InputPortWidth=3  IndexOptions=Index vector (dialog),Index vector (dialog)  Indices=3,3  OutputSizes=1,1
  Sqrt1 : Sqrt  Commented=on
  Sum5 : Sum  Commented=on  Inputs=++++
  qerr : Outport
  wires:
  A_I2B_err/1 -> Mapping choice/1(A_I2B_err1)
  Mapping choice/1(q_err) -> qerr/1  "q_err"
  Gain2/1 -> From q4/1(q4)  "q4"
  Selector11/1 -> Sum5/4
  Sum5/1 -> Sqrt1/1
  Constant1/1 -> Sum5/1
  Selector10/1 -> Sum5/3
  Selector/1 -> Sum5/2
  Sqrt1/1 -> Gain2/1

== system ADCS_orbiter_detumbling/Sensor and Attitude Determination/Subsystem4 ==
  A_I2B_err : Inport
  Discrete Derivative : simulink/Discrete/Discrete Derivative  gainval=1.0  ICPrevScaledInput=0.0  OutMin=[]  OutMax=[]  OutDataType=fixdt(1, 16)  OutScaling=2^-10  DoSatur=off
  Gain : Gain  Gain=-1
  Matrix Multiply : Product  Multiplication=Matrix(*)
  Scope : Scope  NumInputPorts=2
  Selector : Selector  NumberOfDimensions=2  InputPortWidth=3  IndexOptions=Index vector (dialog),Index vector (dialog)  Indices=3,2  OutputSizes=1,1
  Selector1 : Selector  NumberOfDimensions=2  InputPortWidth=3  IndexOptions=Index vector (dialog),Index vector (dialog)  Indices=1,3  OutputSizes=1,1
  Selector2 : Selector  NumberOfDimensions=2  InputPortWidth=3  IndexOptions=Index vector (dialog),Index vector (dialog)  Indices=2,1  OutputSizes=1,1
  Transpose : Math  Operator=transpose
  Vector Concatenate : Concatenate  NumInputs=3
  w_err_DCM : Outport
  wires:
  Vector Concatenate/1 -> w_err_DCM/1
  Selector2/1 -> Vector Concatenate/3
  Selector1/1 -> Vector Concatenate/2
  Selector/1 -> Vector Concatenate/1
  Gain/1 -> Selector/1, Selector1/1, Selector2/1
  Matrix Multiply/1 -> Gain/1
  Discrete Derivative/1 -> Scope/2, Matrix Multiply/1
  Transpose/1 -> Scope/1, Matrix Multiply/2
  A_I2B_err/1 -> Discrete Derivative/1, Transpose/1

== system ADCS_orbiter_detumbling/Actuators/Subsystem/If Action Subsystem ==
  In1 : Inport
  Action Port : ActionPort  ActionPortLabel=if(u1 > F_max)
  Out1 : Outport
  wires:
  In1/1 -> Out1/1

== system ADCS_orbiter_detumbling/Actuators/Subsystem/If Action Subsystem1 ==
  In1 : Inport
  Action Port : ActionPort  ActionPortLabel=elseif(u1<F_min)
  Out1 : Outport
  wires:
  In1/1 -> Out1/1

== system ADCS_orbiter_detumbling/Actuators/Subsystem/If Action Subsystem2 ==
  In1 : Inport
  Action Port : ActionPort  ActionPortLabel=else
  Out1 : Outport
  wires:
  In1/1 -> Out1/1

== system ADCS_orbiter_detumbling/Actuators/Subsystem1/If Action Subsystem ==
  In1 : Inport
  Action Port : ActionPort  ActionPortLabel=if(u1 > F_max)
  Out1 : Outport
  wires:
  In1/1 -> Out1/1

== system ADCS_orbiter_detumbling/Actuators/Subsystem1/If Action Subsystem1 ==
  In1 : Inport
  Action Port : ActionPort  ActionPortLabel=elseif(u1<F_min)
  Out1 : Outport
  wires:
  In1/1 -> Out1/1

== system ADCS_orbiter_detumbling/Actuators/Subsystem1/If Action Subsystem2 ==
  In1 : Inport
  Action Port : ActionPort  ActionPortLabel=else
  Out1 : Outport
  wires:
  In1/1 -> Out1/1

== system ADCS_orbiter_detumbling/Actuators/Subsystem10/If Action Subsystem ==
  In1 : Inport
  Action Port : ActionPort  ActionPortLabel=if(u1 > 0)
  Out2 : Outport
  wires:
  In1/1 -> Out2/1

== system ADCS_orbiter_detumbling/Actuators/Subsystem10/If Action Subsystem1 ==
  In1 : Inport
  Input : Inport  Port=2
  Input1 : Inport  Port=3
  Action Port : ActionPort  ActionPortLabel=else
  If : If  NumInputs=2  IfExpression=u1 > 0 & u2==0
  If Action Subsystem : Subsystem  TreatAsAtomicUnit=on
  If Action Subsystem1 : Subsystem  TreatAsAtomicUnit=on
  Merge : Merge
  Out1 : Outport
  wires:
  In1/1 -> If Action Subsystem1/1(In1)
  Input/1 -> If/1  "u(k-1)"
  Input1/1 -> If/2  "u(k-2)"
  If/1 -> If Action Subsystem/Action
  If/2 -> If Action Subsystem1/Action
  If Action Subsystem1/1(Out1) -> Merge/2
  If Action Subsystem/1(Out1) -> Merge/1
  Merge/1 -> Out1/1

== system ADCS_orbiter_detumbling/Actuators/Subsystem11/If Action Subsystem ==
  In1 : Inport
  Action Port : ActionPort  ActionPortLabel=if(u1 > 0)
  Out2 : Outport
  wires:
  In1/1 -> Out2/1

== system ADCS_orbiter_detumbling/Actuators/Subsystem11/If Action Subsystem1 ==
  In1 : Inport
  Input : Inport  Port=2
  Input1 : Inport  Port=3
  Action Port : ActionPort  ActionPortLabel=else
  If : If  NumInputs=2  IfExpression=u1 > 0 & u2==0
  If Action Subsystem : Subsystem  TreatAsAtomicUnit=on
  If Action Subsystem1 : Subsystem  TreatAsAtomicUnit=on
  Merge : Merge
  Out1 : Outport
  wires:
  Merge/1 -> Out1/1
  If Action Subsystem/1(Out1) -> Merge/1
  If Action Subsystem1/1(Out1) -> Merge/2
  If/2 -> If Action Subsystem1/Action
  If/1 -> If Action Subsystem/Action
  Input1/1 -> If/2  "u(k-2)"
  Input/1 -> If/1  "u(k-1)"
  In1/1 -> If Action Subsystem1/1(In1)

== system ADCS_orbiter_detumbling/Actuators/Subsystem12/If Action Subsystem ==
  In1 : Inport
  Action Port : ActionPort  ActionPortLabel=if(u1 > 0)
  Out2 : Outport
  wires:
  In1/1 -> Out2/1

== system ADCS_orbiter_detumbling/Actuators/Subsystem12/If Action Subsystem1 ==
  In1 : Inport
  Input : Inport  Port=2
  Input1 : Inport  Port=3
  Action Port : ActionPort  ActionPortLabel=else
  If : If  NumInputs=2  IfExpression=u1 > 0 & u2==0
  If Action Subsystem : Subsystem  TreatAsAtomicUnit=on
  If Action Subsystem1 : Subsystem  TreatAsAtomicUnit=on
  Merge : Merge
  Out1 : Outport
  wires:
  In1/1 -> If Action Subsystem1/1(In1)
  Input/1 -> If/1  "u(k-1)"
  Input1/1 -> If/2  "u(k-2)"
  If/1 -> If Action Subsystem/Action
  If/2 -> If Action Subsystem1/Action
  If Action Subsystem1/1(Out1) -> Merge/2
  If Action Subsystem/1(Out1) -> Merge/1
  Merge/1 -> Out1/1

== system ADCS_orbiter_detumbling/Actuators/Subsystem13/If Action Subsystem ==
  In1 : Inport
  Action Port : ActionPort  ActionPortLabel=if(u1 > 0)
  Out2 : Outport
  wires:
  In1/1 -> Out2/1

== system ADCS_orbiter_detumbling/Actuators/Subsystem13/If Action Subsystem1 ==
  In1 : Inport
  Input : Inport  Port=2
  Input1 : Inport  Port=3
  Action Port : ActionPort  ActionPortLabel=else
  If : If  NumInputs=2  IfExpression=u1 > 0 & u2==0
  If Action Subsystem : Subsystem  TreatAsAtomicUnit=on
  If Action Subsystem1 : Subsystem  TreatAsAtomicUnit=on
  Merge : Merge
  Out1 : Outport
  wires:
  Merge/1 -> Out1/1
  If Action Subsystem/1(Out1) -> Merge/1
  If Action Subsystem1/1(Out1) -> Merge/2
  If/2 -> If Action Subsystem1/Action
  If/1 -> If Action Subsystem/Action
  Input1/1 -> If/2  "u(k-2)"
  Input/1 -> If/1  "u(k-1)"
  In1/1 -> If Action Subsystem1/1(In1)

== system ADCS_orbiter_detumbling/Actuators/Subsystem14/If Action Subsystem ==
  In1 : Inport
  Action Port : ActionPort  ActionPortLabel=if(u1 > 0)
  Out2 : Outport
  wires:
  In1/1 -> Out2/1

== system ADCS_orbiter_detumbling/Actuators/Subsystem14/If Action Subsystem1 ==
  In1 : Inport
  Input : Inport  Port=2
  Input1 : Inport  Port=3
  Action Port : ActionPort  ActionPortLabel=else
  If : If  NumInputs=2  IfExpression=u1 > 0 & u2==0
  If Action Subsystem : Subsystem  TreatAsAtomicUnit=on
  If Action Subsystem1 : Subsystem  TreatAsAtomicUnit=on
  Merge : Merge
  Out1 : Outport
  wires:
  In1/1 -> If Action Subsystem1/1(In1)
  Input/1 -> If/1  "u(k-1)"
  Input1/1 -> If/2  "u(k-2)"
  If/1 -> If Action Subsystem/Action
  If/2 -> If Action Subsystem1/Action
  If Action Subsystem1/1(Out1) -> Merge/2
  If Action Subsystem/1(Out1) -> Merge/1
  Merge/1 -> Out1/1

== system ADCS_orbiter_detumbling/Actuators/Subsystem15/If Action Subsystem ==
  In1 : Inport
  Action Port : ActionPort  ActionPortLabel=if(u1 > 0)
  Out2 : Outport
  wires:
  In1/1 -> Out2/1

== system ADCS_orbiter_detumbling/Actuators/Subsystem15/If Action Subsystem1 ==
  In1 : Inport
  Input : Inport  Port=2
  Input1 : Inport  Port=3
  Action Port : ActionPort  ActionPortLabel=else
  If : If  NumInputs=2  IfExpression=u1 > 0 & u2==0
  If Action Subsystem : Subsystem  TreatAsAtomicUnit=on
  If Action Subsystem1 : Subsystem  TreatAsAtomicUnit=on
  Merge : Merge
  Out1 : Outport
  wires:
  Merge/1 -> Out1/1
  If Action Subsystem/1(Out1) -> Merge/1
  If Action Subsystem1/1(Out1) -> Merge/2
  If/2 -> If Action Subsystem1/Action
  If/1 -> If Action Subsystem/Action
  Input1/1 -> If/2  "u(k-2)"
  Input/1 -> If/1  "u(k-1)"
  In1/1 -> If Action Subsystem1/1(In1)

== system ADCS_orbiter_detumbling/Actuators/Subsystem2/If Action Subsystem ==
  In1 : Inport
  Action Port : ActionPort  ActionPortLabel=if(u1 > F_max)
  Out1 : Outport
  wires:
  In1/1 -> Out1/1

== system ADCS_orbiter_detumbling/Actuators/Subsystem2/If Action Subsystem1 ==
  In1 : Inport
  Action Port : ActionPort  ActionPortLabel=elseif(u1<F_min)
  Out1 : Outport
  wires:
  In1/1 -> Out1/1

== system ADCS_orbiter_detumbling/Actuators/Subsystem2/If Action Subsystem2 ==
  In1 : Inport
  Action Port : ActionPort  ActionPortLabel=else
  Out1 : Outport
  wires:
  In1/1 -> Out1/1

== system ADCS_orbiter_detumbling/Actuators/Subsystem3/If Action Subsystem ==
  In1 : Inport
  Action Port : ActionPort  ActionPortLabel=if(u1 > F_max)
  Out1 : Outport
  wires:
  In1/1 -> Out1/1

== system ADCS_orbiter_detumbling/Actuators/Subsystem3/If Action Subsystem1 ==
  In1 : Inport
  Action Port : ActionPort  ActionPortLabel=elseif(u1<F_min)
  Out1 : Outport
  wires:
  In1/1 -> Out1/1

== system ADCS_orbiter_detumbling/Actuators/Subsystem3/If Action Subsystem2 ==
  In1 : Inport
  Action Port : ActionPort  ActionPortLabel=else
  Out1 : Outport
  wires:
  In1/1 -> Out1/1
